simulink model "S_MTET_PROP_MPPT_ALG_V1"  (R2017a)
settings: Solver=FixedStepDiscrete  StartTime=0.0  StopTime=10.0  RelTol=1e-3
undefined symbols (not defined in the file or in its folder): Down, GPTRIP1SEL, GPTRIP2SEL, TZ1, TZ2, Up
libraries: c2802xlib x3, c2806xlib x2
settings Model: ExtModeTrigDuration=8  Creator=dricl  LastModifiedBy=dricl
settings OptimizationCC: DefaultUnderspecifiedDataType=single  PassReuseOutputArgsAs=Individual arguments  MaxStackSize=512
settings DebuggingCC: ParameterTunabilityLossMsg=error
settings HardwareCC: ProdBitPerChar=16  ProdBitPerInt=16  ProdBitPerPointer=32  ProdBitPerSizeT=32  ProdBitPerPtrDiffT=32  ProdLargestAtomicInteger=Integer  ProdLargestAtomicFloat=None  ProdWordSize=16  ProdLongLongMode=on  ProdHWDeviceType=Texas Instruments->C2000
settings SFSimCC: MATLABDynamicMemAlloc=off
settings RTWCC: SystemTargetFile=ert.tlc  HardwareBoard=TI Piccolo F2806x  TLCOptions=-aInlineSetEventsForThisBaseRateFcn=TLC_FALSE -aSuppressMultiTaskScheduler=TLC_FALSE -aRateBasedStepFcn=1  TemplateMakefile=ert_default_tmf  Description=Embedded Coder  Toolchain=Texas Instruments Code Composer Studio v5 (C2000)  CodeExecutionProfiling=on  CodeProfilingSaveOptions=AllData  CodeProfilingInstrumentation=on
settings CodeAppCC: ForceParamTrailComments=on  IgnoreCustomStorageClasses=off  OperatorAnnotations=on  SimulinkDataObjDesc=on  SFDataObjDesc=on  MATLABFcnDesc=on  InsertBlockDesc=on  MATLABSourceComments=on
settings ERTTargetCC: CodeReplacementLibrary=TI C28x  MemSecPackage=tic2000demospkg  MemSecFuncExecute=code_ramfuncs

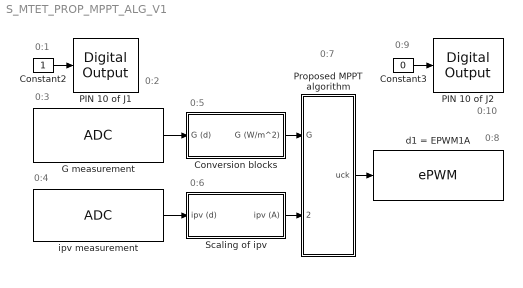
== system S_MTET_PROP_MPPT_ALG_V1 ==
  note: 0:1
  note: 0:2
  note: 0:3
  note: 0:4
  note: 0:5
  note: 0:6
  note: 0:7
  note: 0:8
  note: 0:9
  note: 0:10
  Constant2 : Constant  Priority=1  SampleTime=0.0002
  Constant3 : Constant  Priority=9  Value=0  SampleTime=0.0002
  Conversion blocks : Subsystem  Priority=5  TreatAsAtomicUnit=on
  G measurement : c2802xlib/ADC  Priority=3  ADCModule=1  samplingMode=Single sample mode  ADCResolution=12-bit (Single-ended input)  useSOC1=SOC1  useSOC2=SOC0_SOC1  SOCAcquisitionWindow=7  SOCTriggerSource=ePWM1_ADCSOCA  SOCInterruptTrigger=No ADCINT  Ts=0.0002  dType=uint16  postInterrupt=off  interruptSel=ADCINT1  ADCINTContinuous=on  endma=off  chdma=1  blkParamProc=C2000  conv1=ADCINA1  conv2=ADCINA0 and ADCINB0  conv1_Type4=ADCIN0  conv2_Type4=ADCIN0 and ADCIN1
      settings: SourceProductName=Embedded Coder Support Package for Texas Instruments C2000 Processors
  PIN 10 of J1 : c2806xlib/Digital Output  Priority=2  GPIO_Number=GPIO32~GPIO39  GPIO_Bit0=on  GPIO_BIT0_Toggle=off  GPIO_Bit1=off  GPIO_BIT1_Toggle=off  GPIO_Bit2=off  GPIO_BIT2_Toggle=off  GPIO_Bit3=off  GPIO_BIT3_Toggle=off  GPIO_Bit4=off  GPIO_BIT4_Toggle=off  GPIO_Bit5=off  GPIO_BIT5_Toggle=off  GPIO_Bit6=off  GPIO_BIT6_Toggle=off  GPIO_Bit7=off  GPIO_BIT7_Toggle=off
      settings: SourceProductName=Embedded Coder Support Package for Texas Instruments C2000 Processors  SourceProductBaseCode=TIC2000
  PIN 10 of J2 : c2806xlib/Digital Output  Priority=10  GPIO_Number=GPIO32~GPIO39  GPIO_Bit0=on  GPIO_BIT0_Toggle=off  GPIO_Bit1=off  GPIO_BIT1_Toggle=off  GPIO_Bit2=off  GPIO_BIT2_Toggle=off  GPIO_Bit3=off  GPIO_BIT3_Toggle=off  GPIO_Bit4=off  GPIO_BIT4_Toggle=off  GPIO_Bit5=off  GPIO_BIT5_Toggle=off  GPIO_Bit6=off  GPIO_BIT6_Toggle=off  GPIO_Bit7=off  GPIO_BIT7_Toggle=off
      settings: SourceProductName=Embedded Coder Support Package for Texas Instruments C2000 Processors  SourceProductBaseCode=TIC2000
  Proposed MPPT algorithm : Subsystem  Priority=7
  Scaling of ipv : Subsystem  Priority=6  TreatAsAtomicUnit=on
  d1 = EPWM1A : c2802xlib/ePWM  Priority=8  useModule=ePWM1  ePWMxLINKTBPRD=Not Linked  periodUnits=Clock cycles  timerSource=Specify via dialog  timerPeriod_clk=9000  timerPeriod_sec=0.0001  tbshadow=Counter equals to zero  countingMode=Up-Down  phaseActiveEnable=Disable  phaseDirection=Count down after sync  phaseActive=0  synchronizationEnable=off  dcaevt1Sync=off  dcbevt1Sync=off  synchronizationOption=Disable  clockPrescale=1  HSclockPrescale=1  enswap=off  ePWMxAStatus=on  ePWMxAactionLogic1=Do nothing  ePWMxAactionLogic2=Do nothing  ePWMxAactionLogic3=Clear  ePWMxAactionLogic4=Set  ePWMxAactionLogic5=Do nothing  ePWMxAactionLogic6=Do nothing  ePWMxALoadMode=Load on counter equals to zero (CTR=Zero)  ePWMxACSFenable=off  ePWMxACSFvalue=Forcing disable  ePWMxASFreload=Zero  ePWMxBStatus=off  ePWMxBactionLogic1=Set  ePWMxBactionLogic2=Clear  ePWMxBactionLogic3=Do nothing  ePWMxBactionLogic4=Do nothing  ePWMxBactionLogic5=Clear  ePWMxBactionLogic6=Set  ePWMxBLoadMode=Load on counter equals to zero (CTR=Zero)  ePWMxBCSFenable=off  ePWMxBCSFvalue=Forcing disable  ePWMxBSFreload=Zero  ePWNxBOutWay=off  ePWMxLINKCMPA=Not Linked  CMPAUnits=Clock cycles  CMPASource=Input port  CMPAValue_per=50  CMPAValue_clk=4500  enCMPAshadow=Counter equals to zero  ePWMxLINKCMPB=Not Linked  CMPBUnits=Clock cycles  CMPBSource=Specify via dialog  CMPBValue_per=50  CMPBValue_clk=4500  enCMPBshadow=Counter equals to zero  ePWMxLINKCMPC=Not Linked  CMPCUnits=Clock cycles  CMPCSource=Specify via dialog  CMPCValue_per=50  CMPCValue_clk=32000  enCMPCshadow=Counter equals to zero  ePWMxLINKCMPD=Not Linked  CMPDUnits=Clock cycles  CMPDSource=Specify via dialog  CMPDValue_per=50  CMPDValue_clk=32000  enCMPDshadow=Counter equals to zero  enableDBePWMxA=on  enableDBePWMxB=on  enhalfcycle=off  DBpolarity=Active high complementary (AHC)  DBedgeDelay=Positive  DBSource_ePWMxA=ePWMxA  DBSource_ePWMxB=ePWMxA  DBperiodSource=Specify via dialog  REDperiod=50  FEDperiod=50  adcstartModuleA=on  adcrequestEventA=First event  adcstartEventA=Counter equals to period (CTR=PRD)  adcstartEventA_type2=Digital Compare Module A Event 1 start of conversion (DCAEVT1.soc)  adcstartModuleB=off  adcrequestEventB=First event  adcstartEventB=Counter equals to zero (CTR=Zero)  adcstartEventB_type2=Counter equals to zero (CTR=Zero)  intEn=off  intPrd=First event  intSel=Counter equals to zero (CTR=Zero)  intSel_type2=Counter equals to zero (CTR=Zero)  hrpe=off  enHRPWM=off  HRPWM_LoadMode=Counter equals to period (CTR=PRD)  HRPWM_CTLMode=Duty or Period control mode  HRPWM_EDGMode=Both edge  hrpeb=off  enHRPWMB=off  HRPWM_LoadModeB=Counter equals to zero (CTR=ZERO)  HRPWM_CTLModeB=Duty or Period control mode  HRPWM_EDGModeB=Both edge  enSFO=on  enautoconv=on  chopperEnable=off  chopperFrequency=1  chopperFirstwidth=1  chopperDuty=12.5%  tripZonesource=Specify via dialog  tzselOSHT1=off  tzselOSHT2=off  tzselOSHT3=off  tzselOSHDCAEV1=off  tzselOSHDCBEV1=off  tzselCBC1=off  tzselCBC2=off  tzselCBC3=off  tzselCBCDCAEV2=off  tzselCBCDCBEV2=off  tzselOSHT4=off  tzselOSHT5=off  tzselOSHT6=off  tzselCBC4=off  tzselCBC5=off  tzselCBC6=off  enTzOstIntr=off  enTzCbcIntr=off  enTzDCAEVT1Intr=off  enTzDCAEVT2Intr=off  enTzDCBEVT1Intr=off  enTzDCBEVT2Intr=off  ePWMxAforced=No action  ePWMxBforced=No action  DCAEVT1forced=No action  DCBEVT1forced=No action  DCAEVT2forced=No action  DCBEVT2forced=No action  dcah=Trip Zone 1 input (TZ1)  dcal=Trip Zone 2 input (TZ2)  dcbh=Trip Zone 1 input (TZ1)  dcbl=Trip Zone 2 input (TZ2)  dcah_type2=GPTRIP1SEL/(TZ1)  dcal_type2=GPTRIP2SEL/(TZ2)  dcbh_type2=GPTRIP1SEL/(TZ1)  dcbl_type2=GPTRIP2SEL/(TZ2)  gendcaevt1=Event disabled  gendcaevt2=Event disabled  gendcbevt1=Event disabled  gendcbevt2=Event disabled  dcaevt1src=DCAEVT1 with sync  dcaevt2src=DCAEVT2 with sync  dcbevt1src=DCBEVT1 with sync  dcbevt2src=DCBEVT2 with sync  pulsesel=Counter equals to zero (CTR=Zero)  blankinv=off  blankoffset=0  blankwidth=0  evsrcsel=Filtered version of DCAEVT1 (DCAEVT1FILT)  encape=off  PwmType=C2000
      settings: SourceProductName=Embedded Coder Support Package for Texas Instruments C2000 Processors
  ipv measurement : c2802xlib/ADC  Priority=4  ADCModule=1  samplingMode=Single sample mode  ADCResolution=12-bit (Single-ended input)  useSOC1=SOC2  useSOC2=SOC0_SOC1  SOCAcquisitionWindow=7  SOCTriggerSource=ePWM1_ADCSOCA  SOCInterruptTrigger=No ADCINT  Ts=0.0002  dType=uint16  postInterrupt=off  interruptSel=ADCINT1  ADCINTContinuous=on  endma=off  chdma=1  blkParamProc=C2000  conv1=ADCINA0  conv2=ADCINA0 and ADCINB0  conv1_Type4=ADCIN0  conv2_Type4=ADCIN0 and ADCIN1
      settings: SourceProductName=Embedded Coder Support Package for Texas Instruments C2000 Processors
  wires:
  Scaling of ipv/1(ipv (A)) -> Proposed MPPT algorithm/2(x1 = ipv)
  ipv measurement/1 -> Scaling of ipv/1(ipv (d))
  Conversion blocks/1(G (W/m^2)) -> Proposed MPPT algorithm/1(G)
  G measurement/1 -> Conversion blocks/1(G (d))
  Constant2/1 -> PIN 10 of J1/1
  Constant3/1 -> PIN 10 of J2/1
  Proposed MPPT algorithm/1(uck) -> d1 = EPWM1A/1

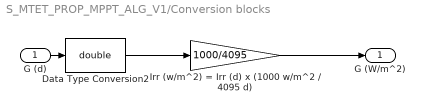
== system S_MTET_PROP_MPPT_ALG_V1/Conversion blocks ==
  G (d) : Inport
  Data Type Conversion2 : DataTypeConversion  OutDataTypeStr=double
  Irr (w/m^2) = Irr (d) x (1000 w/m^2 / 4095 d) : Gain  Gain=1000/4095
  G (W/m^2) : Outport
  wires:
  G (d)/1 -> Data Type Conversion2/1
  Data Type Conversion2/1 -> Irr (w/m^2) = Irr (d) x (1000 w/m^2 / 4095 d)/1
  Irr (w/m^2) = Irr (d) x (1000 w/m^2 / 4095 d)/1 -> G (W/m^2)/1

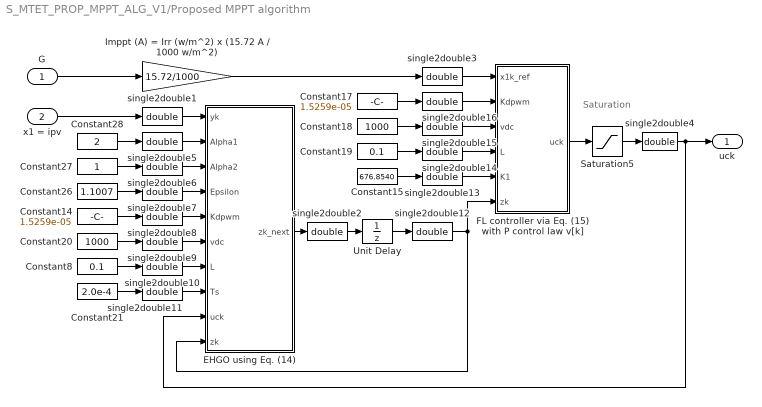
== system S_MTET_PROP_MPPT_ALG_V1/Proposed MPPT algorithm ==
  note: Saturation
  G : Inport
  x1 = ipv : Inport  Port=2
  Constant14 : Constant  Value=1.5259e-05  SampleTime=2.0e-4
  Constant15 : Constant  Value=676.8540  SampleTime=2.0e-4
  Constant17 : Constant  Value=1.5259e-05  SampleTime=2.0e-4
  Constant18 : Constant  Value=1000  SampleTime=2.0e-4
  Constant19 : Constant  Value=0.1  SampleTime=2.0e-4
  Constant20 : Constant  Value=1000  SampleTime=2.0e-4
  Constant21 : Constant  Value=2.0e-4  SampleTime=2.0e-4
  Constant26 : Constant  Value=1.1007  SampleTime=2.0e-4
  Constant27 : Constant  SampleTime=2.0e-4
  Constant28 : Constant  Value=2  SampleTime=2.0e-4
  Constant8 : Constant  Value=0.1  SampleTime=2.0e-4
  EHGO using Eq. (14) : MATLAB Function  TreatAsAtomicUnit=on
  FL controller via Eq. (15) with P control law v[k] : MATLAB Function  TreatAsAtomicUnit=on
  "Imppt (A) = Irr (w/m^2) x (15.72 A / 1000 w/m^2) " : Gain  Gain=15.72/1000
  Saturation5 : Saturate  UpperLimit=9000*0.98  LowerLimit=9000*0.05
  Unit Delay : UnitDelay  SampleTime=2.0e-4
  single2double{1..16} (16 alike) : DataTypeConversion  OutDataTypeStr=double
  uck : Outport
  wires:
  x1 = ipv/1 -> single2double1/1
  G/1 -> "Imppt (A) = Irr (w/m^2) x (15.72 A / 1000 w/m^2) "/1
  FL controller via Eq. (15) with P control law v[k]/1(uck) -> Saturation5/1
  single2double3/1 -> FL controller via Eq. (15) with P control law v[k]/1(x1k_ref)
  single2double1/1 -> EHGO using Eq. (14)/1(yk)
  Saturation5/1 -> single2double4/1
  single2double4/1 -> EHGO using Eq. (14)/9(uck), uck/1
  Constant28/1 -> single2double5/1
  single2double5/1 -> EHGO using Eq. (14)/2(Alpha1)
  Constant27/1 -> single2double6/1
  single2double6/1 -> EHGO using Eq. (14)/3(Alpha2)
  Constant26/1 -> single2double7/1
  single2double7/1 -> EHGO using Eq. (14)/4(Epsilon)
  Constant14/1 -> single2double8/1
  single2double8/1 -> EHGO using Eq. (14)/5(Kdpwm)
  Constant20/1 -> single2double9/1
  single2double9/1 -> EHGO using Eq. (14)/6(vdc)
  Constant8/1 -> single2double10/1
  single2double10/1 -> EHGO using Eq. (14)/7(L)
  Constant21/1 -> single2double11/1
  single2double11/1 -> EHGO using Eq. (14)/8(Ts)
  EHGO using Eq. (14)/1(zk_next) -> single2double2/1
  single2double2/1 -> Unit Delay/1
  Unit Delay/1 -> single2double12/1
  single2double12/1 -> FL controller via Eq. (15) with P control law v[k]/6(zk), EHGO using Eq. (14)/10(zk)
  Constant15/1 -> single2double13/1
  Constant19/1 -> single2double14/1
  Constant18/1 -> single2double15/1
  Constant17/1 -> single2double16/1
  single2double16/1 -> FL controller via Eq. (15) with P control law v[k]/2(Kdpwm)
  single2double15/1 -> FL controller via Eq. (15) with P control law v[k]/3(vdc)
  single2double14/1 -> FL controller via Eq. (15) with P control law v[k]/4(L)
  single2double13/1 -> FL controller via Eq. (15) with P control law v[k]/5(K1)
  "Imppt (A) = Irr (w/m^2) x (15.72 A / 1000 w/m^2) "/1 -> single2double3/1

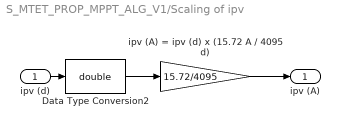
== system S_MTET_PROP_MPPT_ALG_V1/Scaling of ipv ==
  ipv (d) : Inport
  Data Type Conversion2 : DataTypeConversion  OutDataTypeStr=double
  ipv (A) = ipv (d) x (15.72 A / 4095 d) : Gain  Gain=15.72/4095
  ipv (A) : Outport
  wires:
  ipv (d)/1 -> Data Type Conversion2/1
  Data Type Conversion2/1 -> ipv (A) = ipv (d) x (15.72 A / 4095 d)/1
  ipv (A) = ipv (d) x (15.72 A / 4095 d)/1 -> ipv (A)/1

== matlab function S_MTET_PROP_MPPT_ALG_V1/Proposed MPPT algorithm/EHGO using Eq. (14) ==
  data: yk input; Alpha1 input; Alpha2 input; Epsilon input; Kdpwm input; vdc input; L input; Ts input; uck input; zk input; zk_next output
function zk_next = fcn(yk, Alpha1, Alpha2, Epsilon, Kdpwm, vdc, L, Ts, uck, zk)
zk_next = zeros(2,1);
zk_next(1) = zk(1) + Ts*(zk(2)+((Kdpwm/L)*vdc)*uck+ (Alpha1/(Epsilon*Ts))*(yk-zk(1)));
zk_next(2) = zk(2) + Ts*((Alpha2/(Epsilon^2*Ts^2))*(yk-zk(1)));

== matlab function S_MTET_PROP_MPPT_ALG_V1/Proposed MPPT algorithm/FL controller via Eq. (15) with P control law v[k] ==
  data: x1k_ref input; Kdpwm input; vdc input; L input; K1 input; uck output; zk input
function uck = fcn(x1k_ref, Kdpwm, vdc, L, K1, zk)
uck=(L/(Kdpwm*vdc))*(-zk(2)+(-K1*(zk(1)-x1k_ref)));
